simulink model "rotacional_simulink"  (R2023a)
settings: Solver=VariableStepAuto  StartTime=0.0  StopTime=10.0  MaxStep=0.01  RelTol=1e-3
values from neighbouring files (symbols this model uses):
  k = 100    [mov_rotacional.m]    (also in parametros_rotacional.m)
  m = 10    [mov_rotacional.m]    (also in parametros_rotacional.m)
settings Model: Creator=penqu  LastModifiedBy=penqu

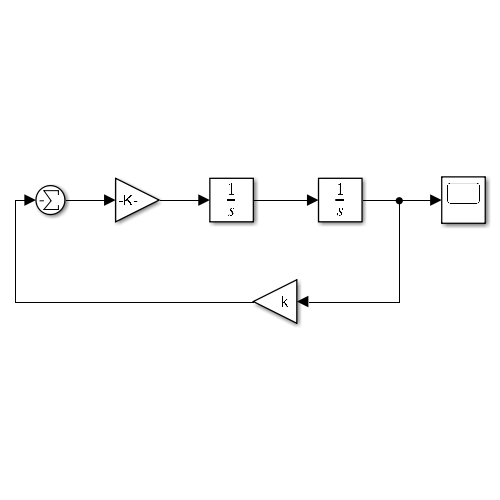
[thumbnail: Simulink's stored preview of the top-level diagram]
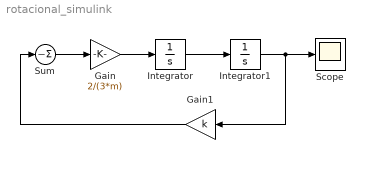
== system rotacional_simulink ==
  Gain : Gain  Gain=2/(3*m)
  Gain1 : Gain  Gain=k
  Integrator : Integrator  InitialCondition=2
  Integrator1 : Integrator
  Scope : Scope
  Sum : Sum  Inputs=-
  wires:
  Gain/1 -> Integrator/1
  Integrator/1 -> Integrator1/1
  Gain1/1 -> Sum/1
  Sum/1 -> Gain/1
  Integrator1/1 -> Gain1/1, Scope/1
